simulink model "arduino_failure_pedal"  (R2021a)
settings: Solver=FixedStepDiscrete  StartTime=0.0  StopTime=10.0  FixedStep=1e-3  RelTol=1e-3
undefined symbols (not defined in the file or in its folder): APP_Modes
settings Model: SILPILModeSetting=veronly  ExtModeTrigDuration=2  Creator=Beshary  LastModifiedBy=Beshary
settings OptimizationCC: DefaultParameterBehavior=Inlined  UseDivisionForNetSlopeComputation=on  GainParamInheritBuiltInType=on  UseFloatMulNetSlope=on  InlineInvariantSignals=on  PassReuseOutputArgsAs=Individual arguments  ZeroExternalMemoryAtStartup=off  ZeroInternalMemoryAtStartup=off  NoFixptDivByZeroProtection=on  EfficientFloat2IntCast=on  LifeSpan=1  MaxStackSize=64  OptimizeBlockOrder=speed  DifferentSizesBufferReuse=on  EfficientTunableParamExpr=on
settings DebuggingCC: ParameterTunabilityLossMsg=error
settings HardwareCC: ProdBitPerInt=16  ProdBitPerPointer=16  ProdBitPerSizeT=16  ProdBitPerPtrDiffT=16  ProdLargestAtomicFloat=None  ProdWordSize=8  ProdLongLongMode=on  ProdHWDeviceType=Atmel->AVR
settings SFSimCC: MATLABDynamicMemAlloc=off
settings RTWCC: SystemTargetFile=ert.tlc  HardwareBoard=Arduino Uno  TemplateMakefile=ert_default_tmf  Toolchain=Arduino AVR  BuildConfiguration=Faster Runs
settings CodeAppCC: ForceParamTrailComments=on  IgnoreCustomStorageClasses=off  OperatorAnnotations=on  SimulinkDataObjDesc=on  SFDataObjDesc=on  CustomSymbolStrGlobalVar=rt$N$M  CustomSymbolStrType=$N$M  CustomSymbolStrFcn=$N$M$F  CustomSymbolStrMacro=$N$M  InsertBlockDesc=on
settings ERTTargetCC: IncludeMdlTerminateFcn=off  CombineSignalStateStructs=on  SuppressErrorStatus=on  SupportAbsoluteTime=off  SupportComplex=off  ExtModeStaticAllocSize=250  InlinedParameterPlacement=NonHierarchical  ERTFilePackagingFormat=CompactWithDataFile

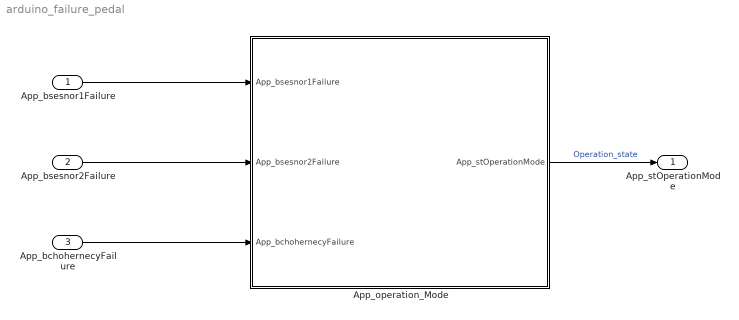
== system arduino_failure_pedal ==
  App_bsesnor1Failure : Inport
  App_bsesnor2Failure : Inport  Port=2
  App_bchohernecyFailure : Inport  Port=3
  App_operation_Mode : Subsystem
      mask DialogControl DescGroupVar Prompt: block
  App_stOperationMode : Outport
  wires:
  App_bsesnor1Failure/1 -> App_operation_Mode/1(App_bsesnor1Failure)
  App_bsesnor2Failure/1 -> App_operation_Mode/2(App_bsesnor2Failure)
  App_bchohernecyFailure/1 -> App_operation_Mode/3(App_bchohernecyFailure)
  App_operation_Mode/1(App_stOperationMode) -> App_stOperationMode/1  "Operation_state"

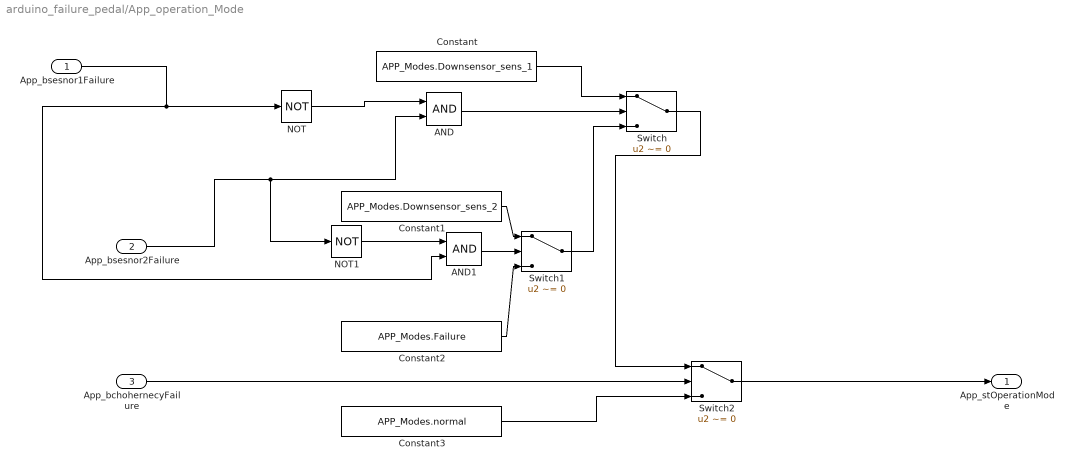
== system arduino_failure_pedal/App_operation_Mode ==
  App_bsesnor1Failure : Inport
  App_bsesnor2Failure : Inport  Port=2
  App_bchohernecyFailure : Inport  Port=3
  AND : Logic  AllPortsSameDT=off  OutDataTypeStr=boolean
  AND1 : Logic  AllPortsSameDT=off  OutDataTypeStr=boolean
  Constant : Constant  Value=APP_Modes.Downsensor_sens_1
  Constant1 : Constant  Value=APP_Modes.Downsensor_sens_2
  Constant2 : Constant  Value=APP_Modes.Failure
  Constant3 : Constant  Value=APP_Modes.normal
  NOT : Logic  Operator=NOT  AllPortsSameDT=off  OutDataTypeStr=boolean
  NOT1 : Logic  Operator=NOT  AllPortsSameDT=off  OutDataTypeStr=boolean
  Switch : Switch  Criteria=u2 ~= 0
  Switch1 : Switch  Criteria=u2 ~= 0
  Switch2 : Switch  Criteria=u2 ~= 0
  App_stOperationMode : Outport  OutDataTypeStr=Enum: APP_Modes
  wires:
  NOT/1 -> AND/1
  App_bsesnor1Failure/1 -> NOT/1, AND1/2
  App_bsesnor2Failure/1 -> NOT1/1, AND/2
  AND/1 -> Switch/2
  Constant/1 -> Switch/1
  NOT1/1 -> AND1/1
  AND1/1 -> Switch1/2
  Constant1/1 -> Switch1/1
  Constant2/1 -> Switch1/3
  App_bchohernecyFailure/1 -> Switch2/2
  Switch/1 -> Switch2/1
  Constant3/1 -> Switch2/3
  Switch2/1 -> App_stOperationMode/1
  Switch1/1 -> Switch/3
